simulink model "new_model_with_vdp"  (R2018b)
settings: Solver=VariableStepAuto  StartTime=0.0  StopTime=10.0  RelTol=1e-3
undefined symbols (not defined in the file or in its folder): Mu, x1_0, x2_0
libraries: simulink x1
settings Model: Creator=kekatos  LastModifiedBy=kekatos

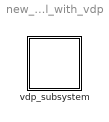
== system new_model_with_vdp ==
  vdp_subsystem : Subsystem

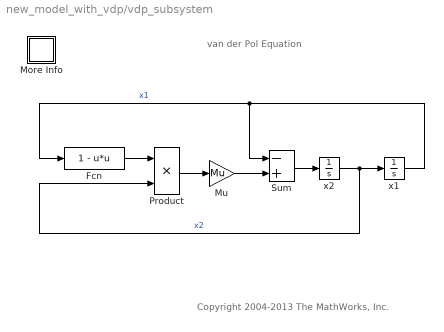
== system new_model_with_vdp/vdp_subsystem ==
  note: van der Pol Equation
  note: Copyright 2004-2013 The MathWorks, Inc.
  Fcn : Fcn  Expr=1 - u*u
  More Info : Subsystem
      mask Display: disp('?')
  Mu : Gain  Gain=Mu  SaturateOnIntegerOverflow=on  OutDataTypeStr=Inherit: Same as input  ParamDataTypeStr=Inherit: Same as input
  Product : Product  SaturateOnIntegerOverflow=on  RndMeth=Zero  InputSameDT=on  OutDataTypeStr=Inherit: Same as first input
  Sum : Sum  Inputs=-+  SaturateOnIntegerOverflow=on  InputSameDT=on  OutDataTypeStr=Inherit: Same as first input
  x1 : Integrator  InitialCondition=x1_0
  x2 : Integrator  InitialCondition=x2_0
  wires:
  Sum/1 -> x2/1
  x2/1 -> x1/1, Product/2  "x2"
  x1/1 -> Sum/1, Fcn/1  "x1"
  Product/1 -> Mu/1
  Mu/1 -> Sum/2
  Fcn/1 -> Product/1

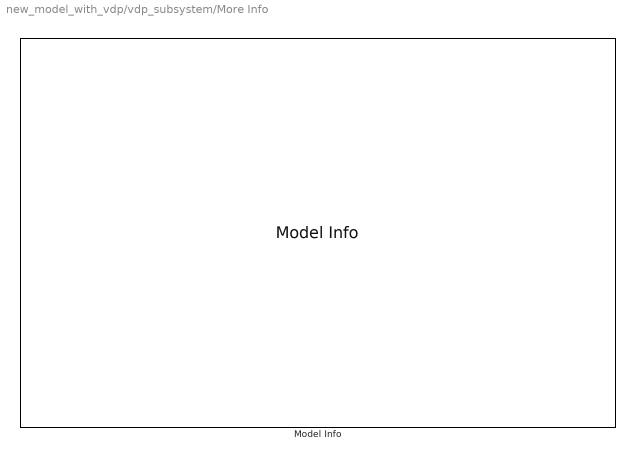
== system new_model_with_vdp/vdp_subsystem/More Info ==
  Model Info : simulink/Model-Wide Utilities/Model Info  BlockCM=None  Frame=on  DisplayStringWithTags=|  HorizontalTextAlignment=Left  LeftAlignmentValue=0.02  SourceBlockDiagram=vdp  TagMaxNumber=20
      | Model Description:
      | -------------------
      | 
      | %<Description>
